simulink model "LQR_probleme_de_urmarire"  (R2023b)
settings: Solver=VariableStepAuto  StartTime=0.0  StopTime=200  RelTol=1e-3
values from neighbouring files (symbols this model uses):
  A = [0 lambda 0 0 ... (first row only)    [rotary_inverted_pendulum.m]    (also in sis_liniar.m)
  B = [0; B21; 0; B41]./lambda    [rotary_inverted_pendulum.m]    (also in sis_liniar.m)
  C = [0 0 1 0]    [rotary_inverted_pendulum.m]
  K = lqr(A,B,Q,R)    [rotary_inverted_pendulum.m]
  N = -inv(C*inv(A-B*K)*B)    [rotary_inverted_pendulum.m]
settings Model: Creator=ovidiuceoca  LastModifiedBy=ovidiuceoca

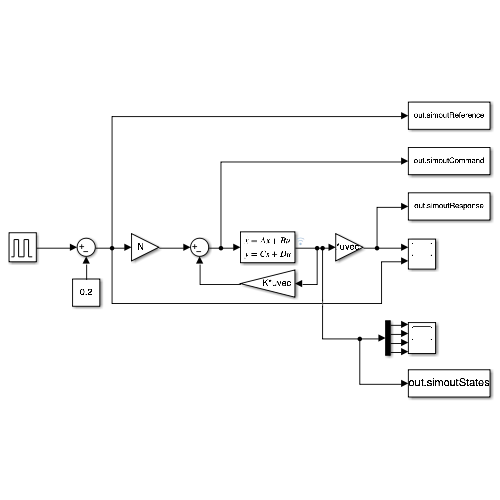
[thumbnail: Simulink's stored preview of the top-level diagram]
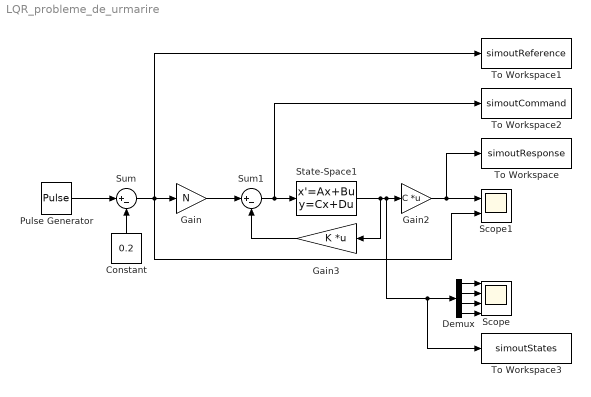
== system LQR_probleme_de_urmarire ==
  Constant : Constant  Value=0.2
  Demux : Demux
  Gain : Gain  Gain=N
  Gain2 : Gain  Gain=C  Multiplication=Matrix(K*u) (u vector)
  Gain3 : Gain  Gain=K  Multiplication=Matrix(K*u) (u vector)
  Pulse Generator : DiscretePulseGenerator  PulseType=Time based  Amplitude=0.4  Period=30  PulseWidth=50  PhaseDelay=15
  Scope : Scope  NumInputPorts=4
  Scope1 : Scope  NumInputPorts=2
  State-Space1 : StateSpace  A=A  B=B  C=eye(4)  D=[0;0;0;0]  InitialCondition=[0;0;20;0]
  Sum : Sum  Inputs=|+-
  Sum1 : Sum  Inputs=|+-
  To Workspace : ToWorkspace  VariableName=simoutResponse  SaveFormat=Timeseries  SampleTime=-1
  To Workspace1 : ToWorkspace  VariableName=simoutReference  SaveFormat=Timeseries  SampleTime=-1
  To Workspace2 : ToWorkspace  VariableName=simoutCommand  SaveFormat=Timeseries  SampleTime=-1
  To Workspace3 : ToWorkspace  VariableName=simoutStates  SaveFormat=Timeseries  SampleTime=-1
  wires:
  Sum/1 -> To Workspace1/1, Scope1/2, Gain/1
  Gain3/1 -> Sum1/2
  Gain/1 -> Sum1/1
  Gain2/1 -> To Workspace/1, Scope1/1
  Pulse Generator/1 -> Sum/1
  Sum1/1 -> To Workspace2/1, State-Space1/1
  Constant/1 -> Sum/2
  State-Space1/1 -> Gain3/1, To Workspace3/1, Demux/1, Gain2/1
  Demux/1 -> Scope/1
  Demux/2 -> Scope/2
  Demux/3 -> Scope/3
  Demux/4 -> Scope/4
